simulink model "sim1"  (R2024b)
settings: Solver=VariableStepAuto  StartTime=0.0  StopTime=20.0  RelTol=1e-3
settings Model: Creator=ether  LastModifiedBy=ether

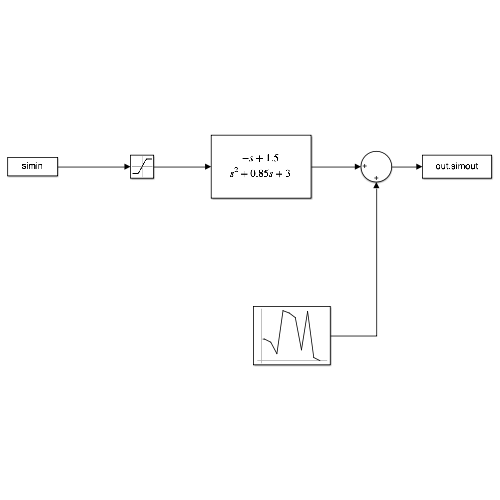
[thumbnail: Simulink's stored preview of the top-level diagram]
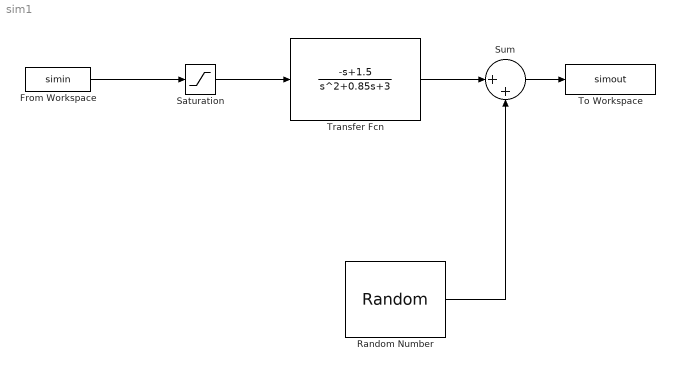
== system sim1 ==
  From Workspace : FromWorkspace  VariableName=simin
  Random Number : RandomNumber  Variance=0.015  SampleTime=0.1
  Saturation : Saturate  UpperLimit=0.9  LowerLimit=-0.9
  Sum : Sum  Inputs=|++
  To Workspace : ToWorkspace  VariableName=simout  SaveFormat=Timeseries  SampleTime=-1
  Transfer Fcn : TransferFcn  Numerator=[-1 1.5]  Denominator=[1 0.85 3]
  wires:
  Saturation/1 -> Transfer Fcn/1
  From Workspace/1 -> Saturation/1
  Transfer Fcn/1 -> Sum/1
  Random Number/1 -> Sum/2
  Sum/1 -> To Workspace/1
